simulink model "Doppelpendel_LQR_2014b"  (R2014b)
settings: Solver=ode15s  StartTime=0.0  StopTime=5
values from neighbouring files (symbols this model uses):
  parLQR = LQR_Entwurf(sysd,parLQR)    [A2_3.m]
  Quantisierung = 1    [LoadParameter.m]
undefined symbols (not defined in the file or in its folder): parDP
libraries: cstblocks x3
settings Model: CovSFcnEnable=on  Creator=tg  LastModifiedBy=jens
settings DataIOCC: SignalLoggingSaveFormat=ModelDataLogs
settings OptimizationCC: ExpressionDepthLimit=2147483647  InitFltsAndDblsToZero=on
settings DebuggingCC: UnderspecifiedInitializationDetection=Classic  MergeDetectMultiDrivingBlocksExec=none  FcnCallInpInsideContextMsg=UseLocalSettings  FrameProcessingCompatibilityMsg=error  StateNameClashWarn=warning
settings SFSimCC: SimParseCustomCode=off
settings GRTTargetCC: CombineOutputUpdateFcns=off  GRTInterface=on

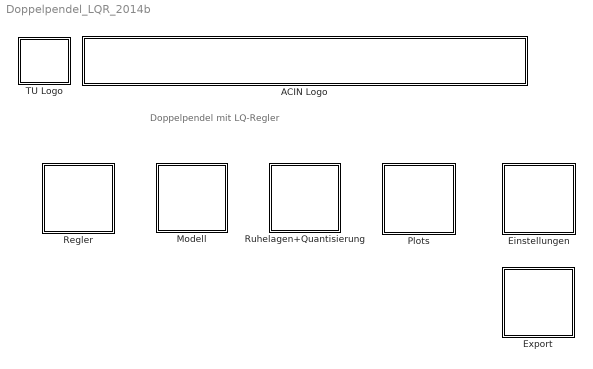
== system Doppelpendel_LQR_2014b ==
  note: Doppelpendel mit LQ-Regler
  ACIN Logo : Subsystem
      mask init:
      | s = get_param(gcb,'UserData');
      mask Display:
      | image(s.logo,[0 0 439 45]);
      | %axis image
  Einstellungen : Subsystem
  Export : Subsystem
  Modell : Subsystem
  Plots : Subsystem
  Regler : Subsystem
  Ruhelagen+Quantisierung : Subsystem
  TU Logo : Subsystem
      mask init:
      | s = get_param(gcb,'UserData');
      mask Display: image(s.logo,[0 0 45 45]);

== system Doppelpendel_LQR_2014b/ACIN Logo ==

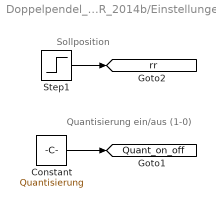
== system Doppelpendel_LQR_2014b/Einstellungen ==
  note: Sollposition
  note: Quantisierung ein/aus (1-0)
  Constant : Constant  Value=Quantisierung
  Step1 : Step  Time=5  After=1*0.1  SampleTime=parLQR.Ta
  tag scope: Quant_on_off=global, rr=global
  wires:
  Step1/1 -> [rr]
  Constant/1 -> [Quant_on_off]

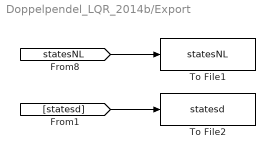
== system Doppelpendel_LQR_2014b/Export ==
  To File1 : ToFile  Filename=statesNL  MatrixName=data  SampleTime=parDP.Ta
  To File2 : ToFile  Filename=statesd  MatrixName=data  SampleTime=parDP.Ta
  wires:
  [statesNL] -> To File1/1
  [statesd] -> To File2/1

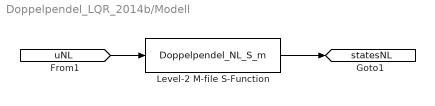
== system Doppelpendel_LQR_2014b/Modell ==
  Level-2 M-file S-Function : M-S-Function  FunctionName=Doppelpendel_NL_S_m  Parameters=parDP.phi10,parDP.omega10,parDP.phi20,parDP.omega20,parDP.s0,parDP.w0,parDP.l1,parDP.l2,parDP.a1,parDP.a2,parDP.m1,parDP.m2,parDP.J1,parDP.J2,parDP.d1,parDP.d2
  tag scope: statesNL=global
  wires:
  [uNL] -> Level-2 M-file S-Function/1
  Level-2 M-file S-Function/1 -> [statesNL]

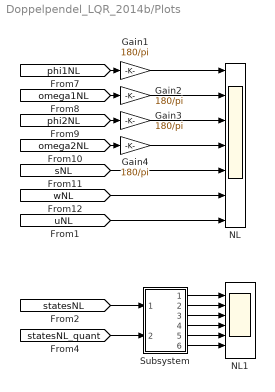
== system Doppelpendel_LQR_2014b/Plots ==
  Gain{1..4} (4 alike) : Gain  Gain=180/pi
  NL : Scope  NumInputPorts=7
      settings: TimeRange=10  MaxDataPoints=5000  SaveToWorkspace=off  SaveName=ScopeData2  YMin=-7.48169~-69.90343~-3.26294~-23.00811~-0.09384~-0.79403~-13.67949  YMax=10.2063~95.20856~3.43872~18.70435~0.13841~0.80195~15.57378  SampleTime=-1
  NL1 : Scope  NumInputPorts=6
      settings: TimeRange=6  MaxDataPoints=5000  SaveToWorkspace=off  YMin=-9.02203~-77.78757~-3.30272~-17.3687~-0.13321~-0.67856  YMax=7.36865~59.56793~3.2598~21.66072~0.13162~0.71451  SampleTime=-1
  Subsystem : Subsystem
  wires:
  [omega1NL] -> Gain2/1
  [omega2NL] -> Gain4/1
  [sNL] -> NL/5
  [wNL] -> NL/6
  Gain1/1 -> NL/1
  Gain2/1 -> NL/2
  Gain3/1 -> NL/3
  Gain4/1 -> NL/4
  [phi1NL] -> Gain1/1
  [phi2NL] -> Gain3/1
  [statesNL] -> Subsystem/1(In1)
  [statesNL_quant] -> Subsystem/2(In2)
  Subsystem/1(Out1) -> NL1/1
  Subsystem/2(Out2) -> NL1/2
  Subsystem/3(Out3) -> NL1/3
  Subsystem/4(Out4) -> NL1/4
  Subsystem/5(Out5) -> NL1/5
  Subsystem/6(Out6) -> NL1/6
  [uNL] -> NL/7

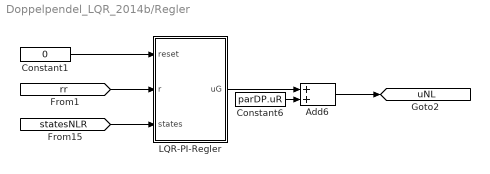
== system Doppelpendel_LQR_2014b/Regler ==
  Add6 : Sum
  Constant1 : Constant  Value=0
  Constant6 : Constant  Value=parDP.uR
  LQR-PI-Regler : MATLAB Function  TreatAsAtomicUnit=on
      settings: PermitHierarchicalResolution=ParametersOnly
  tag scope: uNL=global
  wires:
  Constant6/1 -> Add6/2
  Add6/1 -> [uNL]
  LQR-PI-Regler/1(uG) -> Add6/1
  [statesNLR] -> LQR-PI-Regler/3(states)
  [rr] -> LQR-PI-Regler/2(r)
  Constant1/1 -> LQR-PI-Regler/1(reset)

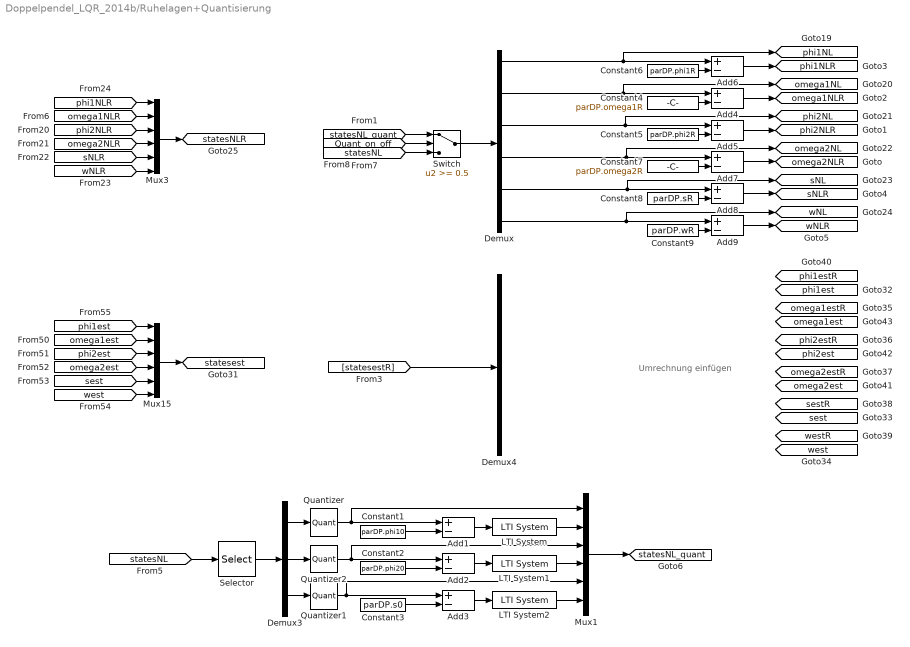
== system Doppelpendel_LQR_2014b/Ruhelagen+Quantisierung ==
  note: Umrechnung
      | einfügen
  Add{1..9} (9 alike) : Sum  Inputs=+-
  Constant1 : Constant  Value=parDP.phi10
  Constant2 : Constant  Value=parDP.phi20
  Constant3 : Constant  Value=parDP.s0
  Constant4 : Constant  Value=parDP.omega1R
  Constant5 : Constant  Value=parDP.phi2R
  Constant6 : Constant  Value=parDP.phi1R
  Constant7 : Constant  Value=parDP.omega2R
  Constant8 : Constant  Value=parDP.sR
  Constant9 : Constant  Value=parDP.wR
  Demux : Demux  Outputs=6
  Demux3 : Demux  Outputs=3
  Demux4 : Demux  Outputs=6
  LTI System : cstblocks/LTI System  sys=Fd_diff  IC=[]
  LTI System1 : cstblocks/LTI System  sys=Fd_diff  IC=[]
  LTI System2 : cstblocks/LTI System  sys=Fd_diff  IC=[]
  Mux1 : Mux  Inputs=6
  Mux15 : Mux  Inputs=6
  Mux3 : Mux  Inputs=6
  Quantizer : Quantizer  QuantizationInterval=Phiquantisierung  SampleTime=parLQR.Ta
  Quantizer1 : Quantizer  QuantizationInterval=Wegquantisierung  SampleTime=parLQR.Ta
  Quantizer2 : Quantizer  QuantizationInterval=Phiquantisierung  SampleTime=parLQR.Ta
  Selector : Selector  InputPortWidth=6  IndexOptions=Index vector (dialog)  Indices=[1 3 5]  OutputSizes=1
  Switch : Switch  Threshold=0.5
  tag scope: omega1NL=global, omega1NLR=global, omega1est=global, omega1estR=global, omega2NL=global, omega2NLR=global, omega2est=global, omega2estR=global, phi1NL=global, phi1NLR=global, phi1est=global, phi1estR=global, phi2NL=global, phi2NLR=global, phi2est=global, phi2estR=global, sNL=global, sNLR=global, sest=global, sestR=global, statesNLR=global, statesNL_quant=global, statesest=global, wNL=global, wNLR=global, west=global, westR=global
  wires:
  [phi1NLR] -> Mux3/1
  [omega1NLR] -> Mux3/2
  [phi2NLR] -> Mux3/3
  [omega2NLR] -> Mux3/4
  [sNLR] -> Mux3/5
  [wNLR] -> Mux3/6
  Mux3/1 -> [statesNLR]
  [phi1est] -> Mux15/1
  [omega1est] -> Mux15/2
  [phi2est] -> Mux15/3
  [omega2est] -> Mux15/4
  [sest] -> Mux15/5
  [west] -> Mux15/6
  Mux15/1 -> [statesest]
  [statesNL] -> Selector/1
  Selector/1 -> Demux3/1
  Demux3/2 -> Quantizer2/1
  Demux3/1 -> Quantizer/1
  Demux3/3 -> Quantizer1/1
  Mux1/1 -> [statesNL_quant]
  LTI System/1 -> Mux1/2
  LTI System2/1 -> Mux1/6
  LTI System1/1 -> Mux1/4
  Add1/1 -> LTI System/1
  Add2/1 -> LTI System1/1
  Add3/1 -> LTI System2/1
  Constant1/1 -> Add1/2
  Constant2/1 -> Add2/2
  Constant3/1 -> Add3/2
  Quantizer1/1 -> Add3/1, Mux1/5
  Quantizer2/1 -> Add2/1, Mux1/3
  Quantizer/1 -> Add1/1, Mux1/1
  [statesestR] -> Demux4/1
  Switch/1 -> Demux/1
  [statesNL] -> Switch/3
  [Quant_on_off] -> Switch/2
  [statesNL_quant] -> Switch/1
  Demux/1 -> Add6/1, [phi1NL]
  Constant6/1 -> Add6/2
  Add6/1 -> [phi1NLR]
  Constant4/1 -> Add4/2
  Demux/2 -> Add4/1, [omega1NL]
  Constant5/1 -> Add5/2
  Demux/3 -> Add5/1, [phi2NL]
  Constant7/1 -> Add7/2
  Demux/4 -> Add7/1, [omega2NL]
  Constant8/1 -> Add8/2
  Demux/5 -> Add8/1, [sNL]
  Constant9/1 -> Add9/2
  Demux/6 -> Add9/1, [wNL]
  Add4/1 -> [omega1NLR]
  Add5/1 -> [phi2NLR]
  Add7/1 -> [omega2NLR]
  Add8/1 -> [sNLR]
  Add9/1 -> [wNLR]

== system Doppelpendel_LQR_2014b/TU Logo ==

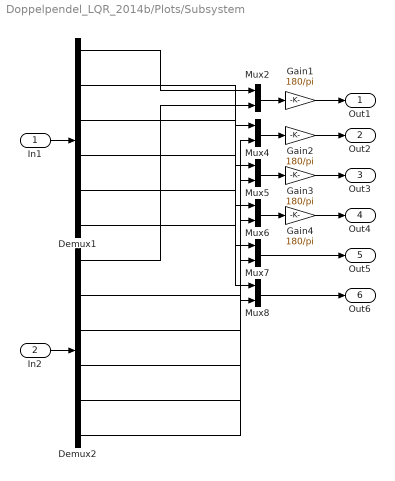
== system Doppelpendel_LQR_2014b/Plots/Subsystem ==
  In1 : Inport
  In2 : Inport  Port=2
  Demux1 : Demux  Outputs=6
  Demux2 : Demux  Outputs=6
  Gain{1..4} (4 alike) : Gain  Gain=180/pi
  Mux{2,4..8} (6 alike) : Mux  Inputs=2
  Out1 : Outport
  Out2 : Outport  Port=2
  Out3 : Outport  Port=3
  Out4 : Outport  Port=4
  Out5 : Outport  Port=5
  Out6 : Outport  Port=6
  wires:
  Demux1/1 -> Mux2/1
  Demux2/1 -> Mux2/2
  Demux2/2 -> Mux4/2
  Demux2/3 -> Mux5/2
  Demux2/4 -> Mux6/2
  Demux2/5 -> Mux7/2
  Demux2/6 -> Mux8/2
  Demux1/6 -> Mux8/1
  Demux1/5 -> Mux7/1
  Demux1/2 -> Mux4/1
  Demux1/3 -> Mux5/1
  Demux1/4 -> Mux6/1
  Mux2/1 -> Gain1/1
  Mux4/1 -> Gain2/1
  In1/1 -> Demux1/1
  Mux5/1 -> Gain3/1
  Mux6/1 -> Gain4/1
  Mux7/1 -> Out5/1
  Mux8/1 -> Out6/1
  In2/1 -> Demux2/1
  Gain1/1 -> Out1/1
  Gain2/1 -> Out2/1
  Gain3/1 -> Out3/1
  Gain4/1 -> Out4/1

== matlab function Doppelpendel_LQR_2014b/Regler/LQR-PI-Regler ==
  settings: updateMethod=DISCRETE  sampleTime=parLQR.Ta
  data: reset input; r input; states input; uG output; parLQR parameter
function uG  = LQR(reset,r,states,parLQR)
%Anfangsbedingung I-Anteil
persistent xI
if isempty(xI) xI = double(0); end
if reset==1 xI = double(0); end

uG = [parLQR.kx parLQR.kI]*[states;xI];
xI = xI+(r-states(5));

end
